simulink model "DiscreteDerivative1"  (R2017b)
settings: Solver=FixedStepDiscrete  StartTime=0.0  StopTime=10.0  FixedStep=0.010000  RelTol=1e-3  EnableMultiTasking=on
libraries: simulink x2
settings Model: Creator=hbourbou  LastModifiedBy=hbourbou
settings DataIOCC: LimitDataPoints=on
settings OptimizationCC: LifeSpan=inf
settings DebuggingCC: SFUnexpectedBacktrackingDiag=warning  SFNoUnconditionalDefaultTransitionDiag=warning  SFExecutionAtInitializationDiag=none
settings HardwareCC: ProdBitPerSizeT=32  ProdBitPerPtrDiffT=32  ProdWordSize=32  ProdHWDeviceType=Specified
settings ModelReferenceCC: PropagateSignalLabelsOutOfModel=off
settings CodeAppCC: StateflowObjectComments=on
settings GRTTargetCC: TargetLangStandard=C89/C90 (ANSI)
settings ConfigComp: CovMetricSettings=dw  CovHtmlReporting=on  CovSaveCumulativeToWorkspaceVar=on  CovSaveSingleToWorkspaceVar=on  CovExternalEMLEnable=off

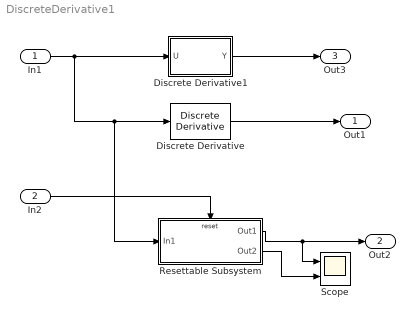
== system DiscreteDerivative1 ==
  In1 : Inport
  In2 : Inport  Port=2
  Discrete Derivative : simulink/Discrete/Discrete Derivative  gainval=1.0  ICPrevScaledInput=3.9  InputProcessing=Inherited  OutMin=[]  OutMax=[]  OutDataType=fixdt(1, 16)  OutScaling=2^-10  DoSatur=off
  Discrete Derivative1 : Subsystem  TreatAsAtomicUnit=on
      settings: MinAlgLoopOccurrences=on
  Resettable Subsystem : Subsystem  TreatAsAtomicUnit=on
  Scope : Scope  NumInputPorts=2
  Out1 : Outport
  Out2 : Outport  Port=2
  Out3 : Outport  Port=3
  wires:
  Discrete Derivative/1 -> Out1/1
  Resettable Subsystem/1(Out1) -> Scope/1, Out2/1
  In2/1 -> Resettable Subsystem/Reset
  In1/1 -> Resettable Subsystem/1(In1), Discrete Derivative/1, Discrete Derivative1/1(U)
  Discrete Derivative1/1(Y) -> Out3/1
  Resettable Subsystem/2(Out2) -> Scope/2

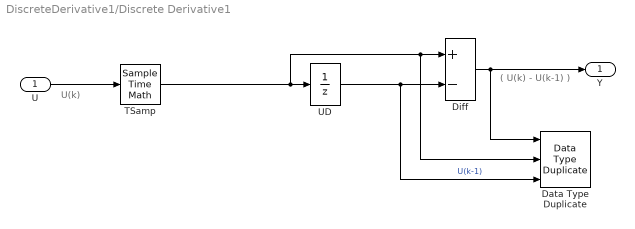
== system DiscreteDerivative1/Discrete Derivative1 ==
  note: ( U(k) - U(k-1) )
  note: U(k)
  U : Inport
  Data Type Duplicate : DataTypeDuplicate  DisableCoverage=on  NumInputPorts=3
  Diff : Sum  Description=Add in CPU  Inputs=+-  OutDataTypeStr=Inherit: Inherit via back propagation
  TSamp : SampleTimeMath  DisableCoverage=on  TsampMathOp=/  weightValue=1  TsampMathImp=Offline Scaling Adjustment
  UD : UnitDelay  Description=Store in Global RAM  DisableCoverage=on  InitialCondition=3.9  SampleTime=-1
  Y : Outport  InitialOutput=0
  wires:
  UD/1 -> Data Type Duplicate/3, Diff/2  "U(k-1)"
  Diff/1 -> Data Type Duplicate/1, Y/1
  TSamp/1 -> Data Type Duplicate/2, Diff/1, UD/1
  U/1 -> TSamp/1

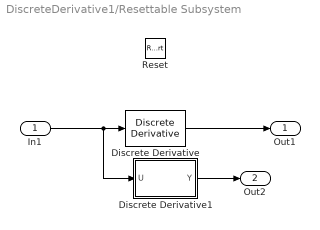
== system DiscreteDerivative1/Resettable Subsystem ==
  In1 : Inport
  Reset : ResetPort  DisableCoverage=on
  Discrete Derivative : simulink/Discrete/Discrete Derivative  gainval=5  ICPrevScaledInput=3.9  InputProcessing=Inherited  OutMin=[]  OutMax=[]  OutDataType=fixdt(1, 16)  OutScaling=2^-10  DoSatur=off
  Discrete Derivative1 : Subsystem  TreatAsAtomicUnit=on
      settings: MinAlgLoopOccurrences=on
  Out1 : Outport
  Out2 : Outport  Port=2
  wires:
  In1/1 -> Discrete Derivative1/1(U), Discrete Derivative/1
  Discrete Derivative/1 -> Out1/1
  Discrete Derivative1/1(Y) -> Out2/1

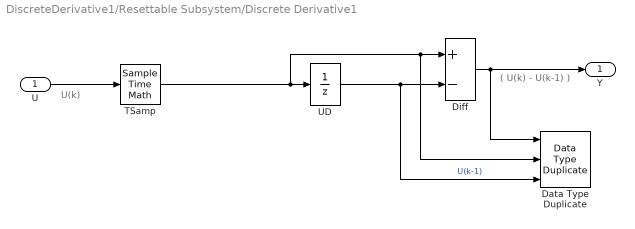
== system DiscreteDerivative1/Resettable Subsystem/Discrete Derivative1 ==
  note: ( U(k) - U(k-1) )
  note: U(k)
  U : Inport
  Data Type Duplicate : DataTypeDuplicate  DisableCoverage=on  NumInputPorts=3
  Diff : Sum  Description=Add in CPU  Inputs=+-  OutDataTypeStr=Inherit: Inherit via back propagation
  TSamp : SampleTimeMath  DisableCoverage=on  TsampMathOp=/  weightValue=1  TsampMathImp=Offline Scaling Adjustment
  UD : UnitDelay  Description=Store in Global RAM  DisableCoverage=on  InitialCondition=3.9  SampleTime=-1
  Y : Outport  InitialOutput=0
  wires:
  UD/1 -> Data Type Duplicate/3, Diff/2  "U(k-1)"
  Diff/1 -> Data Type Duplicate/1, Y/1
  TSamp/1 -> Data Type Duplicate/2, Diff/1, UD/1
  U/1 -> TSamp/1
